simulink model "Airfoil_Read_Data"  (R2016a)
settings: Solver=FixedStepDiscrete  SolverMode=SingleTasking  StartTime=0.0  StopTime=inf  FixedStep=AUTO  RelTol=1e-3
undefined symbols (not defined in the file): serial
libraries: instrumentlib x3, simulink x1, realtime_pacer_lib x1
settings Model: Creator=Tomas  LastModifiedBy=Tomas

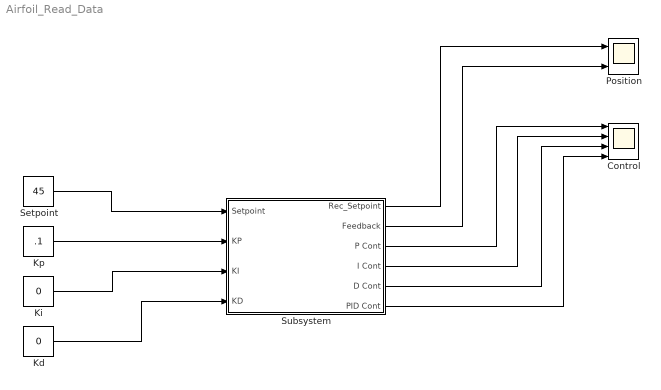
== system Airfoil_Read_Data ==
  Control : Scope  NumInputPorts=4
  Kd : Constant  Value=0  VectorParams1D=off  OutMin=0  OutMax=0.01
  Ki : Constant  Value=0  VectorParams1D=off  OutMin=0  OutMax=5
  Kp : Constant  Value=.1  VectorParams1D=off  OutMin=0  OutMax=1
  Position : Scope  NumInputPorts=2
  Setpoint : Constant  Value=45  VectorParams1D=off  OutMin=-60  OutMax=60
  Subsystem : Subsystem
  wires:
  Ki/1 -> Subsystem/3(KI)
  Kp/1 -> Subsystem/2(KP)
  Setpoint/1 -> Subsystem/1(Setpoint)
  Kd/1 -> Subsystem/4(KD)
  Subsystem/3(P Cont) -> Control/1
  Subsystem/4(I Cont) -> Control/2
  Subsystem/5(D Cont) -> Control/3
  Subsystem/6(PID Cont) -> Control/4
  Subsystem/1(Rec_Setpoint) -> Position/1
  Subsystem/2(Feedback) -> Position/2

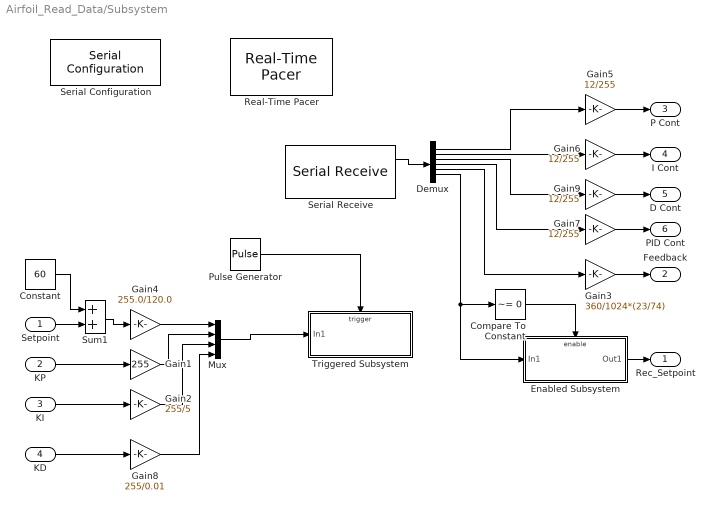
== system Airfoil_Read_Data/Subsystem ==
  Setpoint : Inport
  KP : Inport  Port=2
  KI : Inport  Port=3
  KD : Inport  Port=4
  Compare To Constant : simulink/Logic and Bit Operations/Compare To Constant  relop=~=  const=0  OutDataTypeStr=boolean
  Constant : Constant  Value=60
  Demux : Demux  Outputs=6
  Enabled Subsystem : Subsystem  TreatAsAtomicUnit=on
  Gain1 : Gain  Gain=255  OutDataTypeStr=uint8
  Gain2 : Gain  Gain=255/5  OutDataTypeStr=uint8
  Gain3 : Gain  Gain=360/1024*(23/74)  SaturateOnIntegerOverflow=on
  Gain4 : Gain  Gain=255.0/120.0  OutDataTypeStr=uint8  SaturateOnIntegerOverflow=on
  Gain{5..7,9} (4 alike) : Gain  Gain=12/255
  Gain8 : Gain  Gain=255/0.01  OutDataTypeStr=uint8
  Mux : Mux
  Pulse Generator : DiscretePulseGenerator  PulseType=Time based  Period=0.25  PulseWidth=50  PhaseDelay=2
  Real-Time Pacer : realtime_pacer_lib/Real-Time Pacer  simTimePerRealTime=1
  Serial Configuration : instrumentlib/Serial Configuration  Priority=-200000  ComPortMenu=COM4  ComPort=COM4  ObjConstructor=serial('COM4');  BaudRate=115200  DataBits=8  Parity=none  StopBits=1  FlowControl=none  Timeout=1  ByteOrder=LittleEndian
  Serial Receive : instrumentlib/Serial Receive  ComPortMenu=COM4  ComPort=COM4  ObjConstructor=serial('COM4');  Header=)(  Terminator=<none>  DataSize="[1  6]"  DataType=int16  EnableBlockingMode=off  ActionDataUnavailable=Output last received value  CustomValue=0  SampleTime=.002
  Sum1 : Sum  OutDataTypeStr=int16  SaturateOnIntegerOverflow=on
  Triggered Subsystem : Subsystem  TreatAsAtomicUnit=on
  Rec_Setpoint : Outport
  Feedback : Outport  Port=2
  P Cont : Outport  Port=3
  I Cont : Outport  Port=4
  D Cont : Outport  Port=5
  PID Cont : Outport  Port=6
  wires:
  Serial Receive/1 -> Demux/1
  Gain4/1 -> Mux/1
  Pulse Generator/1 -> Triggered Subsystem/Trigger
  Demux/1 -> Gain5/1
  Demux/2 -> Gain6/1
  Mux/1 -> Triggered Subsystem/1(In1)
  Gain1/1 -> Mux/2
  KP/1 -> Gain1/1
  KI/1 -> Gain2/1
  Gain2/1 -> Mux/3
  Gain5/1 -> P Cont/1
  Gain6/1 -> I Cont/1
  Gain7/1 -> PID Cont/1
  Setpoint/1 -> Sum1/2
  Sum1/1 -> Gain4/1
  Constant/1 -> Sum1/1
  Gain3/1 -> Feedback/1
  KD/1 -> Gain8/1
  Gain8/1 -> Mux/4
  Demux/5 -> Gain3/1
  Demux/4 -> Gain7/1
  Gain9/1 -> D Cont/1
  Demux/3 -> Gain9/1
  Demux/6 -> Compare To Constant/1, Enabled Subsystem/1(In1)
  Enabled Subsystem/1(Out1) -> Rec_Setpoint/1
  Compare To Constant/1 -> Enabled Subsystem/Enable

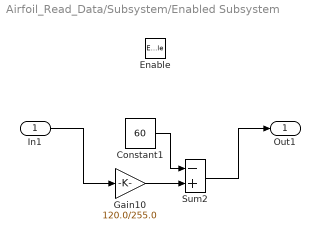
== system Airfoil_Read_Data/Subsystem/Enabled Subsystem ==
  In1 : Inport
  Enable : EnablePort
  Constant1 : Constant  Value=60
  Gain10 : Gain  Gain=120.0/255.0  OutDataTypeStr=double  SaturateOnIntegerOverflow=on
  Sum2 : Sum  Inputs=-+  OutDataTypeStr=double  SaturateOnIntegerOverflow=on
  Out1 : Outport
  wires:
  Constant1/1 -> Sum2/1
  Gain10/1 -> Sum2/2
  Sum2/1 -> Out1/1
  In1/1 -> Gain10/1

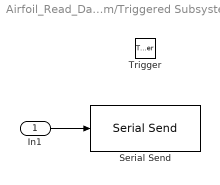
== system Airfoil_Read_Data/Subsystem/Triggered Subsystem ==
  In1 : Inport
  Trigger : TriggerPort  TriggerType=either  VariantControl=Variant
  Serial Send : instrumentlib/Serial Send  ComPortMenu=COM4  ComPort=COM4  ObjConstructor=serial('COM4');  Terminator=<none>  EnableBlockingMode=off
  wires:
  In1/1 -> Serial Send/1
